simulink model "noClueWhatImDoing"  (R2015a)
settings: Solver=FixedStepDiscrete  StartTime=0.0  StopTime=inf  FixedStep=timestep  RelTol=1e-3
libraries: xpcquanserlib x2, simulink x1
settings Model: SimulationMode=external  CovSFcnEnable=off  Creator=Venkatraman  LastModifiedBy=jms6
settings SolverCC: EnableConcurrentExecution=on
settings OptimizationCC: BlockReduction=off  OptimizeBlockIOStorage=off  BufferReuse=off  GlobalBufferReuse=off  ExpressionFolding=off  LocalBlockOutputs=off
settings DebuggingCC: SolverPrmCheckMsg=warning
settings HardwareCC: ProdIntDivRoundTo=Zero  ProdEndianess=LittleEndian  ProdLongLongMode=on  ProdHWDeviceType=Generic->32-bit x86 compatible  TargetLongLongMode=on  TargetIntDivRoundTo=Zero  TargetEndianess=LittleEndian  TargetHWDeviceType=MATLAB Host
settings RTWCC: SystemTargetFile=slrt.tlc  TemplateMakefile=slrt_default_tmf  Description=Simulink Real-Time  RTWVerbose=off  RTWCompilerOptimization=on
settings SimulinkRealTimeCC: GeneratePreprocessorConditionals=Disable all

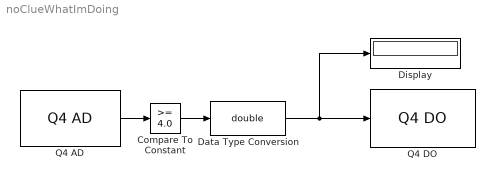
== system noClueWhatImDoing ==
  Compare To Constant : simulink/Logic and Bit Operations/Compare To Constant  relop=>=  const=4.0  OutDataTypeStr=boolean
  Data Type Conversion : DataTypeConversion  OutMin=[0]  OutMax=[1]  OutDataTypeStr=double
  Display : Display
  Q4 AD : xpcquanserlib/A//D/Q4 AD  channel=[1]  sampleTime=0.001  slot=-1
  "Q4 DO " : xpcquanserlib/Digital Output/Q4 DO   channel=[2]  reset=[1]  initValue=[0]  sampleTime=.001  slot=-1
  wires:
  Q4 AD/1 -> Compare To Constant/1
  Compare To Constant/1 -> Data Type Conversion/1
  Data Type Conversion/1 -> Display/1, "Q4 DO "/1
